simulink library "Motor_InductionMachine_lib"  (Simulink 8.1)
settings: Solver=ode45  StartTime=0.0  StopTime=10.0  RelTol=1e-3
undefined symbols (not defined in the file): gcbh, Motor, motor_lib, sps_rtmsupport, Ts
libraries: spsAsynchronousMachineModel x6, powerlib x4, breaker_lib x2
settings Model: Creator=ed12083  LastModifiedBy=g73labuser

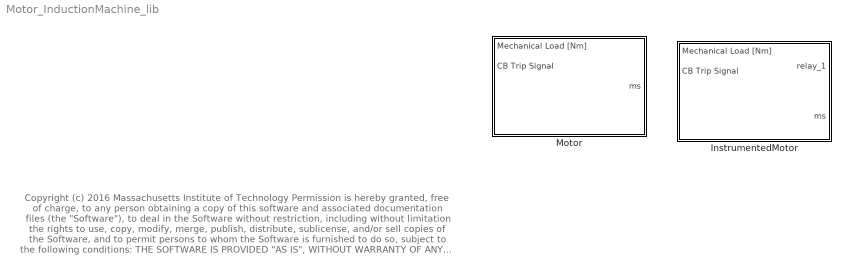
== system Motor_InductionMachine_lib ==
  note: Copyright (c) 2016 Massachusetts Institute of Technology
      | Permission is hereby granted, free of charge, to any person obtaining a copy of this software and associated documentation files (the "Software"), to deal
      | in the Software without restriction, including without limitation the rights to use, copy, modify, merge, publish, distribute, sublicense, and/or sell copies of the
      | Software, and to permit persons to whom the Software is furnished to do so, subject to the following conditions:
      |
      | THE SOFTWARE IS PROVIDED "AS IS", WITHOUT WARRANTY OF ANY KIND, EXPRESS OR IMPLIED, INCLUDING BUT NOT LIMITED TO THE
      | WARRANTIES OF MERCHANTABILITY, FITNESS FOR A PARTICULAR PURPOSE AND NONINFRINGEMENT. IN NO EVENT SHALL THE AUTHORS
      | OR COPYRIGHT HOLDERS BE LIABLE FOR ANY CLAIM, DAMAGES OR OTHER LIABILITY, WHETHER IN AN ACTION OF CONTRACT, TORT OR
      | OTHERWISE, ARISING FROM, OUT OF OR IN CONNECTION WITH THE SOFTWARE OR THE USE OR OTHER DEALINGS IN THE SOFTWARE.
  InstrumentedMotor : Subsystem  AncestorBlock=Motor_InductionMachine_lib/Motor
  Motor : Subsystem  AncestorBlock=motor_lib/Motor

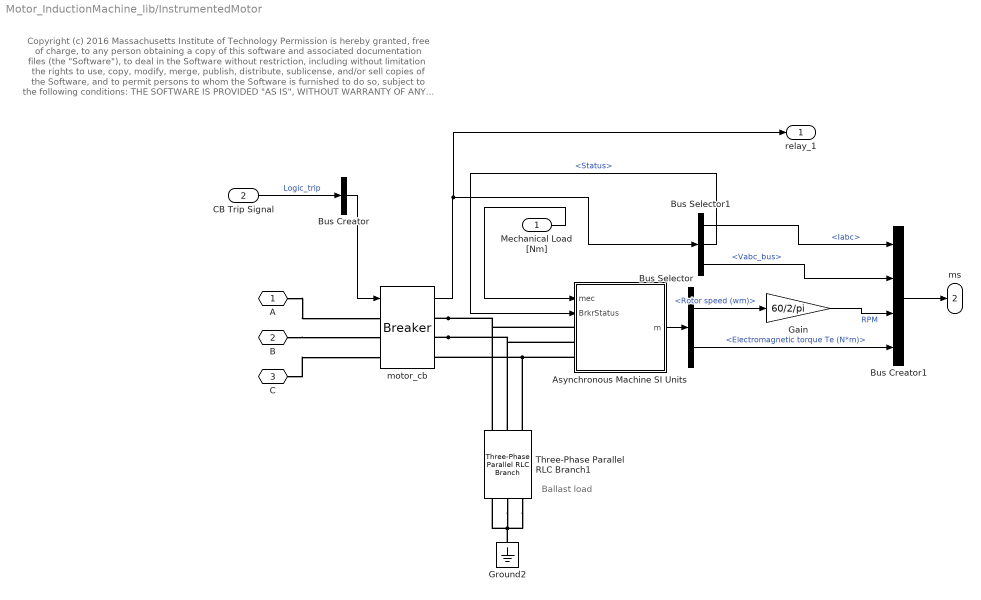
== system Motor_InductionMachine_lib/InstrumentedMotor ==
  note: Ballast load
  note: Copyright (c) 2016 Massachusetts Institute of Technology
      | Permission is hereby granted, free of charge, to any person obtaining a copy of this software and associated documentation files (the "Software"), to deal
      | in the Software without restriction, including without limitation the rights to use, copy, modify, merge, publish, distribute, sublicense, and/or sell copies of the
      | Software, and to permit persons to whom the Software is furnished to do so, subject to the following conditions:
      |
      | THE SOFTWARE IS PROVIDED "AS IS", WITHOUT WARRANTY OF ANY KIND, EXPRESS OR IMPLIED, INCLUDING BUT NOT LIMITED TO THE
      | WARRANTIES OF MERCHANTABILITY, FITNESS FOR A PARTICULAR PURPOSE AND NONINFRINGEMENT. IN NO EVENT SHALL THE AUTHORS
      | OR COPYRIGHT HOLDERS BE LIABLE FOR ANY CLAIM, DAMAGES OR OTHER LIABILITY, WHETHER IN AN ACTION OF  CONTRACT, TORT OR
      | OTHERWISE, ARISING FROM, OUT OF OR IN CONNECTION WITH THE SOFTWARE OR THE USE OR OTHER DEALINGS IN THE SOFTWARE.
  Mechanical Load [Nm] : Inport
  CB Trip Signal : Inport  Port=2
  Asynchronous Machine SI Units : Subsystem  DialogController=POWERSYS.PowerSysDialog  LoadFcn=sps_rtmsupport('LoadFcn',gcbh);  StartFcn=sps_rtmsupport('StartFcn',gcbh);  StopFcn=sps_rtmsupport('StopFcn',gcbh);  mask(Asynchronous Machine){PresetModel=No, MechanicalLoad=Torque Tm, ShowDetailedParameters=on, RotorType=Squirrel-cage, ReferenceFrame=Stationary, NominalParameters=[ 136700/.92/.93, 480, 60 ], Stator=[ 0.029 0.226/377/1.5], Rotor=[ 0.022*3 0.226/377/1.5], Cage1=[ 0.022 0.226/377], Cage2=[ 0.022 0.226/377], Lm=13.04/377, Mechanical=[ 63.87 0  2 ], PolePairs=2, InitialConditions=[1 0 0 0 0 0 0 0], Units=SI, LoadFlowParameters=1492000, SimulateSaturation=off, Saturation=[14.03593122, 27.81365428, 53.79336849, 72.68890987, 97.98006896, 148.6815601, 215.7428561, 302.9841135, 420.4778367 ; 230, 322, 414, 460, 506, 552, 598, 644, 690], TsPowergui=0, TsBlock=-1, IterativeModel=Trapezoidal non iterative, Pmec=0}
      mask prompts: PresetModel "Preset model:"; MechanicalLoad "Mechanical input:"; ShowDetailedParameters "Show detailed parameters"; RotorType "Rotor type:"; ReferenceFrame "Reference frame:"; NominalParameters "Nominal power, voltage (line-line), and frequency [ Pn(VA),Vn(Vrms),fn(Hz) ]:"; Stator "Stator resistance and inductance[ Rs(ohm)  Lls(H) ]:"; Rotor "Rotor resistance and inductance [ Rr'(ohm)  Llr'(H) ]:"; Cage1 "Cage 1 resistance and inductance  [ Rr1' (ohm)  Llr1' (H) ]:"; Cage2 "Cage 2 resistance and inductance  [ Rr2' (ohm)  Llr2' (H) ]:"; Lm "Mutual inductance Lm (H):"; Mechanical "Inertia, friction factor, pole pairs [ J(kg.m^2)  F(N.m.s)   p() ]:"; PolePairs "Pole pairs p ():"; InitialConditions "Initial conditions"; Units "Mask units:"; LoadFlowParameters "Load flow Parameters"; SimulateSaturation "Simulate saturation"; Saturation "Saturation Parameters [i1,i2,... (Arms) ; v1,v2,...(VrmsLL)]"; TsPowergui "Sample time of powergui block"; TsBlock "Sample time (-1 for inherited)"; IterativeModel "Discrete solver model"; Pmec "Mechanical power (W)"
      mask help: Implements a three-phase asynchronous machine (wound rotor, squirrel cage or double squirrel cage) modeled in a selectable dq reference frame (rotor, stator, or synchronous). Stator and rotor windings are connected in wye to an internal neutral point.
      mask init:
      | block = gcb;
      | [Ts,SM,WantBlockChoice,X,Y,txt] = powericon('AsynchronousMachineInit',block,TsPowergui,TsBlock,MechanicalLoad,RotorType,ReferenceFrame,NominalParameters,Stator,Rotor,Cage1,Cage2,Lm,Mechanical,PolePairs,InitialConditions,Units,SimulateSaturation,Saturation,IterativeModel);
      | powericon('SetInternalModels','set',block,WantBlockChoice); sps_rtmsupport('parametereditingmodes',block, [1 2 3 4 5 15 17 21]); 
      | powericon('ShaftInput',(block));
      settings: AttributesFormatString=\n  CopyFcn=sps_rtmsupport('CopyFcn',gcbh); powericon('psbloadfunction',gcbh,'gotofrom','UpdateGotoTag');  DeleteFcn=sps_rtmsupport('DeleteFcn',gcbh);  UndoDeleteFcn=sps_rtmsupport('UndoDeleteFcn',gcbh);  ModelCloseFcn=sps_rtmsupport('ModelCloseFcn',gcbh);  PreSaveFcn=sps_rtmsupport('PreSaveFcn',gcbh);  PostSaveFcn=sps_rtmsupport('PostSaveFcn',gcbh);  NameChangeFcn=sps_rtmsupport('NameChangeFcn',gcbh);  PreCopyFcn=sps_rtmsupport('PreCopyFcn',gcbh);  OpenFcn=sps_rtmsupport('OpenFcn',gcbh, [1 2 3 4 5 15 17 21]);  CloseFcn=sps_rtmsupport('CloseFcn',gcbh);  PreDeleteFcn=sps_rtmsupport('PreDeleteFcn',gcbh);
      mask Help: helpview(psbhelp);
      mask TypeOptions PresetModel: No | 01:  5 HP   460 V 60Hz 1750 RPM            | 02:  10 HP  460 V 60Hz 1760 RPM           | 03:  20 HP  460 V 60Hz 1760 RPM           | 04:  50 HP  460 V 60Hz 1780 RPM           | 05:  100 HP 460 V 60Hz 1780 RPM          | 06:  150 HP 460 V 60Hz 1785 RPM          | 07:  200 HP 460 V 60Hz 1785 RPM          | 08:  5 HP   575 V 60Hz 1750 RPM            | 09:  10 HP  575 V 60Hz 1760 RPM           | 10:  20 HP  575 V 60Hz 1765 RPM           | 11:  50 HP  575 V 60Hz 1775 RPM           | 12:  100 HP 575 V 60Hz 1780 RPM          | 13:  150 HP 575 V 60Hz 1785 RPM          | 14:  200 HP 575 V 60Hz 1785 RPM          | 15:  5.4 HP (4KW)   400 V  50Hz 1430 RPM   | 16:  10 HP (7.5KW)  400 V 50Hz 1440 RPM  | 17:  20 HP (15KW)   400 V 50Hz 1460 RPM   | 18:  50 HP (37KW)   400 V 50Hz 1480 RPM   | 19:  100 HP (75KW)  400 V 50Hz 1484 RPM  | 20:  150 HP (110KW) 400 V 50Hz 1487 RPM | 21:  215 HP (160KW) 400 V 50Hz 1487 RPM
      mask Callback PresetModel: powericon('AsynchronousMachineCback',gcb,'SI');
      mask TypeOptions MechanicalLoad: Torque Tm | Speed w | Mechanical rotational port
      mask Callback MechanicalLoad: %powericon('AsynchronousMachineCback',gcb);
      mask Callback ShowDetailedParameters: %powericon('AsynchronousMachineCback',gcb);
      mask TypeOptions RotorType: Wound | Squirrel-cage | Double squirrel-cage
      mask Callback RotorType: powericon('AsynchronousMachineCback',gcb,'SI','RotorType');
      mask TypeOptions ReferenceFrame: Rotor | Stationary | Synchronous
      mask TypeOptions Units: SI
      mask Callback SimulateSaturation: powericon('AsynchronousMachineCback',gcb,'SI');
      mask TypeOptions IterativeModel: Trapezoidal non iterative | Trapezoidal iterative (alg. loop) | Forward Euler
      mask Callback Pmec: sps_rtmsupport('parametereditingmodes',gcbh, [1 2 3 4 5 15 17 21]);
      mask Display:
      | plot(X.p1,Y.p1,X.p2,Y.p2,X.p3,Y.p3,X.p4,Y.p4,X.p5,Y.p5,X.p6,Y.p6,X.p7,Y.p7,X.p8,Y.p8,X.p9,Y.p9,X.p10,Y.p10)
      | color('blue');
      | plot(X.p11,Y.p11);
      | plot(X.p12,Y.p12);
      | if strcmp(get_param(block,'MechanicalLoad'),'Mechanical rotational port');
      | else
      |     port_label('input',1,SM.PortLabel)
      | end
      | text(0,20,txt,'HorizontalAlignment','Center')
  Bus Creator : BusCreator  Inputs=1
  Bus Creator1 : BusCreator
  Bus Selector : BusSelector  OutputSignals=Mechanical.Rotor speed (wm),Mechanical.Electromagnetic torque Te (N*m)
  Bus Selector1 : BusSelector  OutputSignals=Iabc,Status,Vabc_bus
  Gain : Gain  Gain=60/2/pi
  Ground2 : powerlib/Elements/Ground  LConnTagsString=a
  Three-Phase Parallel RLC Branch1 : powerlib/Elements/Three-Phase Parallel RLC Branch  LConnTagsString=A|B|C  RConnTagsString=A|B|C  BranchType=RC  Resistance=1e6  Inductance=inf  Capacitance=10e-6  Measurements=None
  motor_cb : breaker_lib/Breaker  Ts=Ts
  A : PMIOPort  Port=1  Side=Left
  B : PMIOPort  Port=2  Side=Left
  C : PMIOPort  Port=3  Side=Left
  relay_1 : Outport
  ms : Outport  Port=2
  wires:
  Bus Selector1/2 -> Asynchronous Machine SI Units/2(BrkrStatus)  "<Status>"
  Bus Selector1/1 -> Bus Creator1/1  "<Iabc>"
  Bus Selector1/3 -> Bus Creator1/2  "<Vabc_bus>"
  Bus Creator1/1 -> ms/1
  CB Trip Signal/1 -> Bus Creator/1  "Logic_trip"
  Bus Creator/1 -> motor_cb/1
  Mechanical Load [Nm]/1 -> Asynchronous Machine SI Units/1(mec)
  Asynchronous Machine SI Units/1(m) -> Bus Selector/1
  Bus Selector/1 -> Gain/1  "<Rotor speed (wm)>"
  Bus Selector/2 -> Bus Creator1/4  "<Electromagnetic torque Te (N*m)>"
  Gain/1 -> Bus Creator1/3  "RPM"
  motor_cb/1 -> Bus Selector1/1, relay_1/1
  connections:
  motor_cb/RConn1 -- Three-Phase Parallel RLC Branch1/RConn1 -- Asynchronous Machine SI Units/LConn1
  motor_cb/RConn2 -- Three-Phase Parallel RLC Branch1/RConn2 -- Asynchronous Machine SI Units/LConn2
  Asynchronous Machine SI Units/LConn3 -- motor_cb/RConn3 -- Three-Phase Parallel RLC Branch1/RConn3
  Three-Phase Parallel RLC Branch1/LConn2 -- Three-Phase Parallel RLC Branch1/LConn3 -- Ground2/LConn1 -- Three-Phase Parallel RLC Branch1/LConn1
  A/RConn1 -- motor_cb/LConn1
  B/RConn1 -- motor_cb/LConn2
  C/RConn1 -- motor_cb/LConn3

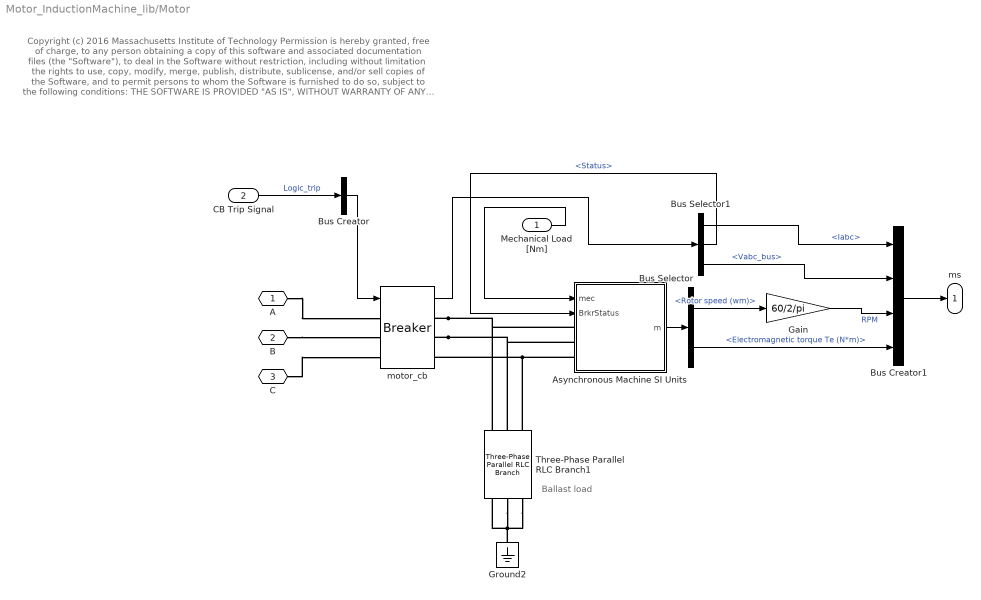
== system Motor_InductionMachine_lib/Motor ==
  note: Ballast load
  note: Copyright (c) 2016 Massachusetts Institute of Technology
      | Permission is hereby granted, free of charge, to any person obtaining a copy of this software and associated documentation files (the "Software"), to deal
      | in the Software without restriction, including without limitation the rights to use, copy, modify, merge, publish, distribute, sublicense, and/or sell copies of the
      | Software, and to permit persons to whom the Software is furnished to do so, subject to the following conditions:
      |
      | THE SOFTWARE IS PROVIDED "AS IS", WITHOUT WARRANTY OF ANY KIND, EXPRESS OR IMPLIED, INCLUDING BUT NOT LIMITED TO THE
      | WARRANTIES OF MERCHANTABILITY, FITNESS FOR A PARTICULAR PURPOSE AND NONINFRINGEMENT. IN NO EVENT SHALL THE AUTHORS
      | OR COPYRIGHT HOLDERS BE LIABLE FOR ANY CLAIM, DAMAGES OR OTHER LIABILITY, WHETHER IN AN ACTION OF CONTRACT, TORT OR
      | OTHERWISE, ARISING FROM, OUT OF OR IN CONNECTION WITH THE SOFTWARE OR THE USE OR OTHER DEALINGS IN THE SOFTWARE.
  Mechanical Load [Nm] : Inport
  CB Trip Signal : Inport  Port=2
  Asynchronous Machine SI Units : Subsystem  DialogController=POWERSYS.PowerSysDialog  LoadFcn=sps_rtmsupport('LoadFcn',gcbh);  StartFcn=sps_rtmsupport('StartFcn',gcbh);  StopFcn=sps_rtmsupport('StopFcn',gcbh);  mask(Asynchronous Machine){PresetModel=No, MechanicalLoad=Torque Tm, ShowDetailedParameters=on, RotorType=Squirrel-cage, ReferenceFrame=Stationary, NominalParameters=[ 136700/.92/.93, 480, 60 ], Stator=[ 0.029 0.226/377/1.5], Rotor=[ 0.022*3 0.226/377/1.5], Cage1=[ 0.022 0.226/377], Cage2=[ 0.022 0.226/377], Lm=13.04/377, Mechanical=[ 63.87 0  2 ], PolePairs=2, InitialConditions=[1 0 0 0 0 0 0 0], Units=SI, LoadFlowParameters=1492000, SimulateSaturation=off, Saturation=[14.03593122, 27.81365428, 53.79336849, 72.68890987, 97.98006896, 148.6815601, 215.7428561, 302.9841135, 420.4778367 ; 230, 322, 414, 460, 506, 552, 598, 644, 690], TsPowergui=0, TsBlock=-1, IterativeModel=Trapezoidal non iterative, Pmec=0}
      mask prompts: PresetModel "Preset model:"; MechanicalLoad "Mechanical input:"; ShowDetailedParameters "Show detailed parameters"; RotorType "Rotor type:"; ReferenceFrame "Reference frame:"; NominalParameters "Nominal power, voltage (line-line), and frequency [ Pn(VA),Vn(Vrms),fn(Hz) ]:"; Stator "Stator resistance and inductance[ Rs(ohm)  Lls(H) ]:"; Rotor "Rotor resistance and inductance [ Rr'(ohm)  Llr'(H) ]:"; Cage1 "Cage 1 resistance and inductance  [ Rr1' (ohm)  Llr1' (H) ]:"; Cage2 "Cage 2 resistance and inductance  [ Rr2' (ohm)  Llr2' (H) ]:"; Lm "Mutual inductance Lm (H):"; Mechanical "Inertia, friction factor, pole pairs [ J(kg.m^2)  F(N.m.s)   p() ]:"; PolePairs "Pole pairs p ():"; InitialConditions "Initial conditions"; Units "Mask units:"; LoadFlowParameters "Load flow Parameters"; SimulateSaturation "Simulate saturation"; Saturation "Saturation Parameters [i1,i2,... (Arms) ; v1,v2,...(VrmsLL)]"; TsPowergui "Sample time of powergui block"; TsBlock "Sample time (-1 for inherited)"; IterativeModel "Discrete solver model"; Pmec "Mechanical power (W)"
      mask help: Implements a three-phase asynchronous machine (wound rotor, squirrel cage or double squirrel cage) modeled in a selectable dq reference frame (rotor, stator, or synchronous). Stator and rotor windings are connected in wye to an internal neutral point.
      mask init: same as Motor_InductionMachine_lib/InstrumentedMotor/Asynchronous Machine SI Units
      settings: AttributesFormatString=\n  CopyFcn=sps_rtmsupport('CopyFcn',gcbh); powericon('psbloadfunction',gcbh,'gotofrom','UpdateGotoTag');  DeleteFcn=sps_rtmsupport('DeleteFcn',gcbh);  UndoDeleteFcn=sps_rtmsupport('UndoDeleteFcn',gcbh);  ModelCloseFcn=sps_rtmsupport('ModelCloseFcn',gcbh);  PreSaveFcn=sps_rtmsupport('PreSaveFcn',gcbh);  PostSaveFcn=sps_rtmsupport('PostSaveFcn',gcbh);  NameChangeFcn=sps_rtmsupport('NameChangeFcn',gcbh);  PreCopyFcn=sps_rtmsupport('PreCopyFcn',gcbh);  OpenFcn=sps_rtmsupport('OpenFcn',gcbh, [1 2 3 4 5 15 17 21]);  CloseFcn=sps_rtmsupport('CloseFcn',gcbh);  PreDeleteFcn=sps_rtmsupport('PreDeleteFcn',gcbh);
      mask Help: helpview(psbhelp);
      mask TypeOptions PresetModel: No | 01:  5 HP   460 V 60Hz 1750 RPM            | 02:  10 HP  460 V 60Hz 1760 RPM           | 03:  20 HP  460 V 60Hz 1760 RPM           | 04:  50 HP  460 V 60Hz 1780 RPM           | 05:  100 HP 460 V 60Hz 1780 RPM          | 06:  150 HP 460 V 60Hz 1785 RPM          | 07:  200 HP 460 V 60Hz 1785 RPM          | 08:  5 HP   575 V 60Hz 1750 RPM            | 09:  10 HP  575 V 60Hz 1760 RPM           | 10:  20 HP  575 V 60Hz 1765 RPM           | 11:  50 HP  575 V 60Hz 1775 RPM           | 12:  100 HP 575 V 60Hz 1780 RPM          | 13:  150 HP 575 V 60Hz 1785 RPM          | 14:  200 HP 575 V 60Hz 1785 RPM          | 15:  5.4 HP (4KW)   400 V  50Hz 1430 RPM   | 16:  10 HP (7.5KW)  400 V 50Hz 1440 RPM  | 17:  20 HP (15KW)   400 V 50Hz 1460 RPM   | 18:  50 HP (37KW)   400 V 50Hz 1480 RPM   | 19:  100 HP (75KW)  400 V 50Hz 1484 RPM  | 20:  150 HP (110KW) 400 V 50Hz 1487 RPM | 21:  215 HP (160KW) 400 V 50Hz 1487 RPM
      mask Callback PresetModel: powericon('AsynchronousMachineCback',gcb,'SI');
      mask TypeOptions MechanicalLoad: Torque Tm | Speed w | Mechanical rotational port
      mask Callback MechanicalLoad: %powericon('AsynchronousMachineCback',gcb);
      mask Callback ShowDetailedParameters: %powericon('AsynchronousMachineCback',gcb);
      mask TypeOptions RotorType: Wound | Squirrel-cage | Double squirrel-cage
      mask Callback RotorType: powericon('AsynchronousMachineCback',gcb,'SI','RotorType');
      mask TypeOptions ReferenceFrame: Rotor | Stationary | Synchronous
      mask TypeOptions Units: SI
      mask Callback SimulateSaturation: powericon('AsynchronousMachineCback',gcb,'SI');
      mask TypeOptions IterativeModel: Trapezoidal non iterative | Trapezoidal iterative (alg. loop) | Forward Euler
      mask Callback Pmec: sps_rtmsupport('parametereditingmodes',gcbh, [1 2 3 4 5 15 17 21]);
      mask Display:
      | plot(X.p1,Y.p1,X.p2,Y.p2,X.p3,Y.p3,X.p4,Y.p4,X.p5,Y.p5,X.p6,Y.p6,X.p7,Y.p7,X.p8,Y.p8,X.p9,Y.p9,X.p10,Y.p10)
      | color('blue');
      | plot(X.p11,Y.p11);
      | plot(X.p12,Y.p12);
      | if strcmp(get_param(block,'MechanicalLoad'),'Mechanical rotational port');
      | else
      |     port_label('input',1,SM.PortLabel)
      | end
      | text(0,20,txt,'HorizontalAlignment','Center')
  Bus Creator : BusCreator  Inputs=1
  Bus Creator1 : BusCreator
  Bus Selector : BusSelector  OutputSignals=Mechanical.Rotor speed (wm),Mechanical.Electromagnetic torque Te (N*m)
  Bus Selector1 : BusSelector  OutputSignals=Iabc,Status,Vabc_bus
  Gain : Gain  Gain=60/2/pi
  Ground2 : powerlib/Elements/Ground  LConnTagsString=a
  Three-Phase Parallel RLC Branch1 : powerlib/Elements/Three-Phase Parallel RLC Branch  LConnTagsString=A|B|C  RConnTagsString=A|B|C  BranchType=RC  Resistance=1e6  Inductance=inf  Capacitance=10e-6  Measurements=None
  motor_cb : breaker_lib/Breaker  Ts=Ts
  A : PMIOPort  Port=1  Side=Left
  B : PMIOPort  Port=2  Side=Left
  C : PMIOPort  Port=3  Side=Left
  ms : Outport
  wires:
  Bus Selector1/2 -> Asynchronous Machine SI Units/2(BrkrStatus)  "<Status>"
  Bus Selector1/1 -> Bus Creator1/1  "<Iabc>"
  Bus Selector1/3 -> Bus Creator1/2  "<Vabc_bus>"
  Bus Creator1/1 -> ms/1
  CB Trip Signal/1 -> Bus Creator/1  "Logic_trip"
  Bus Creator/1 -> motor_cb/1
  Mechanical Load [Nm]/1 -> Asynchronous Machine SI Units/1(mec)
  Asynchronous Machine SI Units/1(m) -> Bus Selector/1
  Bus Selector/1 -> Gain/1  "<Rotor speed (wm)>"
  Bus Selector/2 -> Bus Creator1/4  "<Electromagnetic torque Te (N*m)>"
  Gain/1 -> Bus Creator1/3  "RPM"
  motor_cb/1 -> Bus Selector1/1
  connections:
  motor_cb/RConn1 -- Three-Phase Parallel RLC Branch1/RConn1 -- Asynchronous Machine SI Units/LConn1
  motor_cb/RConn2 -- Three-Phase Parallel RLC Branch1/RConn2 -- Asynchronous Machine SI Units/LConn2
  Asynchronous Machine SI Units/LConn3 -- motor_cb/RConn3 -- Three-Phase Parallel RLC Branch1/RConn3
  Three-Phase Parallel RLC Branch1/LConn2 -- Three-Phase Parallel RLC Branch1/LConn3 -- Ground2/LConn1 -- Three-Phase Parallel RLC Branch1/LConn1
  A/RConn1 -- motor_cb/LConn1
  B/RConn1 -- motor_cb/LConn2
  C/RConn1 -- motor_cb/LConn3

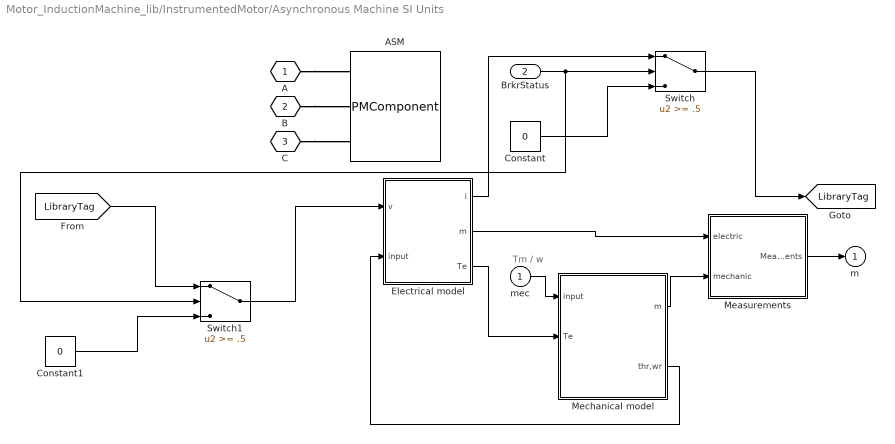
== system Motor_InductionMachine_lib/InstrumentedMotor/Asynchronous Machine SI Units ==
  note: Tm / w
  mec : Inport
  BrkrStatus : Inport  Port=2
  ASM : PMComponent  PhysicalDomain=powersysdomain  LeftPortType=p1  RightPortType=p1  LConnTagsString=A|B|C  RConnTagsString=a|b|c  mask(InnerPowersysBlock){}
  Constant : Constant  Value=0
  Constant1 : Constant  Value=0
  Electrical model : Subsystem  BlockChoice=Continuous
      settings: AttributesFormatString=%<BlockChoice>  TemplateBlock=spsAsynchronousMachineModel/Electrical model  MemberBlocks=Continuous,Continuous double-cage,Discrete,Discrete Trapezoidal,Discrete double-cage,Phasor,Phasor double-cage
  Measurements : Subsystem  BlockChoice=Single-cage SI
      settings: AttributesFormatString=%<BlockChoice>  TemplateBlock=spsAsynchronousMachineModel/Measurements  MemberBlocks=Double-cage SI,Double-cage pu,Single-cage SI,Single-cage pu
  Mechanical model : Subsystem  BlockChoice=Continuous Tm input
      settings: AttributesFormatString=%<BlockChoice>  TemplateBlock=spsAsynchronousMachineModel/Mechanical model  MemberBlocks=Continuous Tm input,Continuous w input,Discrete Tm input,Discrete Tm input Trapezoidal,Discrete w input,Phasor Shaft input,Phasor Tm input,Phasor w input,Shaft input,Shaft input BAL
  Switch : Switch  Threshold=.5
  Switch1 : Switch  Threshold=.5
  A : PMIOPort  Port=1  Side=Left
  B : PMIOPort  Port=2  Side=Left
  C : PMIOPort  Port=3  Side=Left
  m : Outport  InitialOutput=0
  tag scope: LibraryTag=global
  wires:
  Switch1/1 -> Electrical model/1(v)
  Constant1/1 -> Switch1/3
  Switch/1 -> [LibraryTag]
  BrkrStatus/1 -> Switch/2, Switch1/2
  Constant/1 -> Switch/3
  [LibraryTag] -> Switch1/1
  Mechanical model/1(m) -> Measurements/2(mechanic)
  Electrical model/2(m) -> Measurements/1(electric)
  Electrical model/1(i) -> Switch/1
  Measurements/1(Measurements) -> m/1
  Electrical model/3(Te) -> Mechanical model/2(Te)
  mec/1 -> Mechanical model/1(input)
  Mechanical model/2(thr,wr) -> Electrical model/2(input)
  connections:
  C/RConn1 -- ASM/LConn3
  B/RConn1 -- ASM/LConn2
  A/RConn1 -- ASM/LConn1

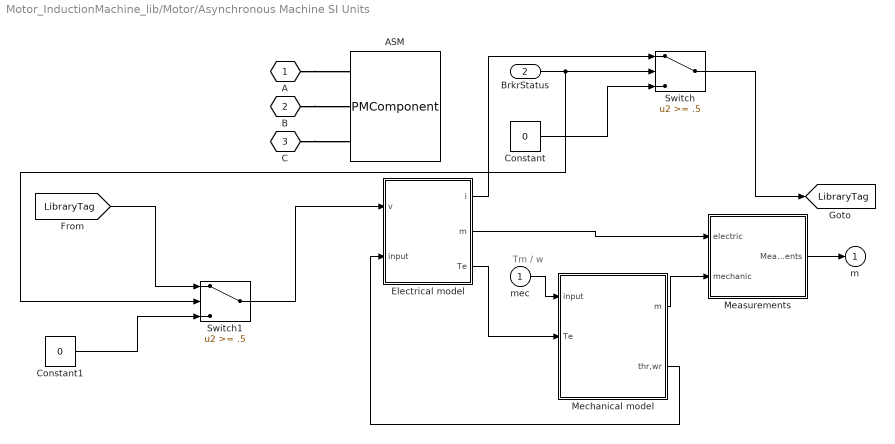
== system Motor_InductionMachine_lib/Motor/Asynchronous Machine SI Units ==
  note: Tm / w
  mec : Inport
  BrkrStatus : Inport  Port=2
  ASM : PMComponent  PhysicalDomain=powersysdomain  LeftPortType=p1  RightPortType=p1  LConnTagsString=A|B|C  RConnTagsString=a|b|c  mask(InnerPowersysBlock){}
  Constant : Constant  Value=0
  Constant1 : Constant  Value=0
  Electrical model : Subsystem  BlockChoice=Continuous
      settings: AttributesFormatString=%<BlockChoice>  TemplateBlock=spsAsynchronousMachineModel/Electrical model  MemberBlocks=Continuous,Continuous double-cage,Discrete,Discrete Trapezoidal,Discrete double-cage,Phasor,Phasor double-cage
  Measurements : Subsystem  BlockChoice=Single-cage SI
      settings: AttributesFormatString=%<BlockChoice>  TemplateBlock=spsAsynchronousMachineModel/Measurements  MemberBlocks=Double-cage SI,Double-cage pu,Single-cage SI,Single-cage pu
  Mechanical model : Subsystem  BlockChoice=Continuous Tm input
      settings: AttributesFormatString=%<BlockChoice>  TemplateBlock=spsAsynchronousMachineModel/Mechanical model  MemberBlocks=Continuous Tm input,Continuous w input,Discrete Tm input,Discrete Tm input Trapezoidal,Discrete w input,Phasor Shaft input,Phasor Tm input,Phasor w input,Shaft input,Shaft input BAL
  Switch : Switch  Threshold=.5
  Switch1 : Switch  Threshold=.5
  A : PMIOPort  Port=1  Side=Left
  B : PMIOPort  Port=2  Side=Left
  C : PMIOPort  Port=3  Side=Left
  m : Outport  InitialOutput=0
  tag scope: LibraryTag=global
  wires:
  Switch1/1 -> Electrical model/1(v)
  Constant1/1 -> Switch1/3
  Switch/1 -> [LibraryTag]
  BrkrStatus/1 -> Switch/2, Switch1/2
  Constant/1 -> Switch/3
  [LibraryTag] -> Switch1/1
  Mechanical model/1(m) -> Measurements/2(mechanic)
  Electrical model/2(m) -> Measurements/1(electric)
  Electrical model/1(i) -> Switch/1
  Measurements/1(Measurements) -> m/1
  Electrical model/3(Te) -> Mechanical model/2(Te)
  mec/1 -> Mechanical model/1(input)
  Mechanical model/2(thr,wr) -> Electrical model/2(input)
  connections:
  C/RConn1 -- ASM/LConn3
  B/RConn1 -- ASM/LConn2
  A/RConn1 -- ASM/LConn1

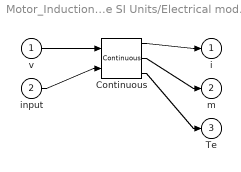
== system Motor_InductionMachine_lib/InstrumentedMotor/Asynchronous Machine SI Units/Electrical model ==
  v : Inport
  input : Inport  Port=2
  Continuous : spsAsynchronousMachineModel/Continuous
  i : Outport
  m : Outport  Port=2
  Te : Outport  Port=3
  wires:
  v/1 -> Continuous/1
  input/1 -> Continuous/2
  Continuous/1 -> i/1
  Continuous/2 -> m/1
  Continuous/3 -> Te/1

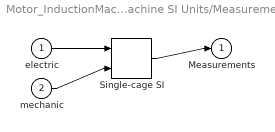
== system Motor_InductionMachine_lib/InstrumentedMotor/Asynchronous Machine SI Units/Measurements ==
  electric : Inport
  mechanic : Inport  Port=2
  Single-cage SI : spsAsynchronousMachineModel/Single-cage SI
  Measurements : Outport
  wires:
  Single-cage SI/1 -> Measurements/1
  mechanic/1 -> Single-cage SI/2
  electric/1 -> Single-cage SI/1

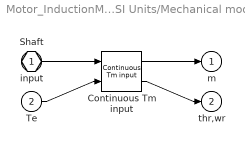
== system Motor_InductionMachine_lib/InstrumentedMotor/Asynchronous Machine SI Units/Mechanical model ==
  input : Inport
  Te : Inport  Port=2
  Continuous Tm input : spsAsynchronousMachineModel/Continuous Tm input
  Shaft : PMIOPort  Port=1  Side=Left
  m : Outport
  thr,wr : Outport  Port=2
  wires:
  input/1 -> Continuous Tm input/1
  Te/1 -> Continuous Tm input/2
  Continuous Tm input/1 -> m/1
  Continuous Tm input/2 -> thr,wr/1

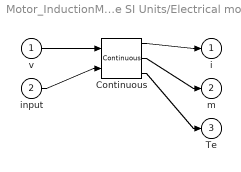
== system Motor_InductionMachine_lib/Motor/Asynchronous Machine SI Units/Electrical model ==
  v : Inport
  input : Inport  Port=2
  Continuous : spsAsynchronousMachineModel/Continuous
  i : Outport
  m : Outport  Port=2
  Te : Outport  Port=3
  wires:
  v/1 -> Continuous/1
  input/1 -> Continuous/2
  Continuous/1 -> i/1
  Continuous/2 -> m/1
  Continuous/3 -> Te/1

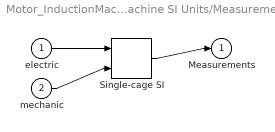
== system Motor_InductionMachine_lib/Motor/Asynchronous Machine SI Units/Measurements ==
  electric : Inport
  mechanic : Inport  Port=2
  Single-cage SI : spsAsynchronousMachineModel/Single-cage SI
  Measurements : Outport
  wires:
  Single-cage SI/1 -> Measurements/1
  mechanic/1 -> Single-cage SI/2
  electric/1 -> Single-cage SI/1

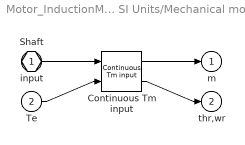
== system Motor_InductionMachine_lib/Motor/Asynchronous Machine SI Units/Mechanical model ==
  input : Inport
  Te : Inport  Port=2
  Continuous Tm input : spsAsynchronousMachineModel/Continuous Tm input
  Shaft : PMIOPort  Port=1  Side=Left
  m : Outport
  thr,wr : Outport  Port=2
  wires:
  input/1 -> Continuous Tm input/1
  Te/1 -> Continuous Tm input/2
  Continuous Tm input/1 -> m/1
  Continuous Tm input/2 -> thr,wr/1
